simulink model "Exp"  (R2017b)
settings: Solver=FixedStepAuto  StartTime=0.0  StopTime=inf  FixedStep=ts  RelTol=1e-3  EnableMultiTasking=on
values from neighbouring files (symbols this model uses):
  acc_gain = 50    [Init_Exp.m]
  cc = 16    [Init_Exp.m]
  channel = 5    [Init_Exp.m]
  f_gait = 0.1    [Init_Exp.m]
  Kg = 80    [Init_Exp.m]
  R_k = diag([1E-4*[1;1];1E-6*[1;1]])    [Init_Exp.m]
  sigma_p = [0.5 1 100000 100000 100000 100000]'    [Init_Exp.m]
  sigma_pp = [sigma sigma sigma sigma sigma sigma]'    [Init_Exp.m]
  sigma_r = [100000 100000 100000 100000]'    [Init_Exp.m]
  sigma_rr = [sigma sigma sigma sigma]'    [Init_Exp.m]
  systemP = [tau_c2,tau_s2,dqs2,eta2,X2,Y2,J2,tau_c1,tau_s1,dqs1,eta1,X1,Y1,J1]    [Init_Exp.m]
  ts = 0.001    [Init_Exp.m]
  vard = vardtimes*1E-2*[2;1]    [Init_Exp.m]
  vardq = 1E-4*[1;1]    [Init_Exp.m]
  varq = 1E-5*[1;1]    [Init_Exp.m]
undefined symbols (not defined in the file or in its folder): acceleration, command, cxk, desired_acc, desired_position, desired_velocity, DiscIntNeverNeededParam, disturbance, immxk, interaction_force, mkxk, motor_torque, observer, position, velocity, xk
libraries: xpcethercatlib x37, slrtlib x9, simulink x1
(part 1 of 2)
settings Model: xpc_rtwmakecfg_data=_xpcethercatlib_  SimulationMode=external  Creator=Admin  LastModifiedBy=Admin
settings SolverCC: ConcurrentTasks=on  AutoInsertRateTranBlk=on
settings DataIOCC: SaveFormat=StructureWithTime
settings OptimizationCC: BlockReduction=off  OptimizeBlockIOStorage=off  BufferReuse=off  GlobalBufferReuse=off  ExpressionFolding=off  LocalBlockOutputs=off
settings HardwareCC: ProdBitPerPointer=32  ProdBitPerSizeT=32  ProdBitPerPtrDiffT=32  ProdLargestAtomicFloat=None  ProdWordSize=32  ProdLongLongMode=on  ProdHWDeviceType=Generic->32-bit x86 compatible
settings RTWCC: SystemTargetFile=slrt.tlc  TemplateMakefile=slrt_default_tmf  Description=Simulink Real-Time  CodeExecutionProfiling=on  RTWCompilerOptimization=on
settings SimulinkRealTimeCC: SupportVariableSizeSignals=on  RL32LogTETModifier=off  xPCConcurrentTasks=on

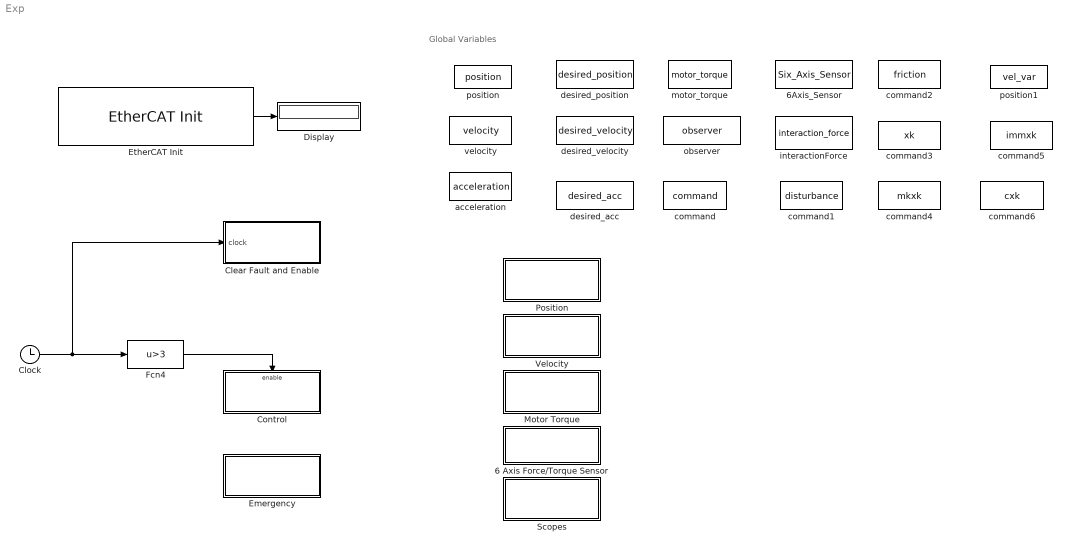
== system Exp ==
  note: Global Variables
  6 Axis Force/Torque Sensor : Subsystem
  6Axis_Sensor : DataStoreMemory  DataStoreName=Six_Axis_Sensor  ReadBeforeWriteMsg=warning  WriteAfterWriteMsg=warning  WriteAfterReadMsg=warning  InitialValue=zeros(12,1)  ShowAdditionalParam=off
  Clear Fault and Enable : Subsystem  TreatAsAtomicUnit=on
  Clock : Clock
  Control : Subsystem  TreatAsAtomicUnit=on
  Display : Display
  Emergency : Subsystem
  "EtherCAT Init " : xpcethercatlib/EtherCAT Init   Priority=0  config_file=D:\lishilei\matlab_workspace\ComputedTorque\GMKMCKF_DOB.xml  device_id=0  pci_bus=2  pci_slot=0  pci_function=0  dctuning=0  enaDebug=off  enaDC=on  errLink=off  masterDbg=off  stateChgDbg=off  baseClock=off  masterCfg=off  logFile='c:\dbglog.txt'  sample_time=0.001000  DCMode=2
      settings: SourceProductName=Simulink Real-Time  SourceProductBaseCode=XP
  Fcn4 : Fcn  Expr=u>3
  Motor Torque : Subsystem
  Position : Subsystem
  Scopes : Subsystem
  Velocity : Subsystem
  acceleration : DataStoreMemory  DataStoreName=acceleration  ReadBeforeWriteMsg=warning  WriteAfterWriteMsg=warning  WriteAfterReadMsg=warning  InitialValue=[0; 0; 0; 0]  ShowAdditionalParam=off
  command : DataStoreMemory  DataStoreName=command  ReadBeforeWriteMsg=warning  WriteAfterWriteMsg=warning  WriteAfterReadMsg=warning  InitialValue=[0; 0; 0; 0]  ShowAdditionalParam=off
  command1 : DataStoreMemory  DataStoreName=disturbance  ReadBeforeWriteMsg=warning  WriteAfterWriteMsg=warning  WriteAfterReadMsg=warning  InitialValue=zeros(4,1)  ShowAdditionalParam=off
  command2 : DataStoreMemory  DataStoreName=friction  ReadBeforeWriteMsg=warning  WriteAfterWriteMsg=warning  WriteAfterReadMsg=warning  InitialValue=[0; 0]  ShowAdditionalParam=off
  command3 : DataStoreMemory  DataStoreName=xk  ReadBeforeWriteMsg=warning  WriteAfterWriteMsg=warning  WriteAfterReadMsg=warning  InitialValue=zeros(6,1)  ShowAdditionalParam=off
  command4 : DataStoreMemory  DataStoreName=mkxk  ReadBeforeWriteMsg=warning  WriteAfterWriteMsg=warning  WriteAfterReadMsg=warning  InitialValue=zeros(6,1)  ShowAdditionalParam=off
  command5 : DataStoreMemory  DataStoreName=immxk  ReadBeforeWriteMsg=warning  WriteAfterWriteMsg=warning  WriteAfterReadMsg=warning  InitialValue=zeros(6,1)  ShowAdditionalParam=off
  command6 : DataStoreMemory  DataStoreName=cxk  ReadBeforeWriteMsg=warning  WriteAfterWriteMsg=warning  WriteAfterReadMsg=warning  InitialValue=zeros(6,1)  ShowAdditionalParam=off
  desired_acc : DataStoreMemory  DataStoreName=desired_acc  ReadBeforeWriteMsg=warning  WriteAfterWriteMsg=warning  WriteAfterReadMsg=warning  InitialValue=[0; 0; 0; 0]  ShowAdditionalParam=off
  desired_position : DataStoreMemory  DataStoreName=desired_position  ReadBeforeWriteMsg=warning  WriteAfterWriteMsg=warning  WriteAfterReadMsg=warning  InitialValue=[0; 0; 0; 0]  ShowAdditionalParam=off
  desired_velocity : DataStoreMemory  DataStoreName=desired_velocity  ReadBeforeWriteMsg=warning  WriteAfterWriteMsg=warning  WriteAfterReadMsg=warning  InitialValue=[0; 0; 0; 0]  ShowAdditionalParam=off
  interactionForce : DataStoreMemory  DataStoreName=interaction_force  ReadBeforeWriteMsg=warning  WriteAfterWriteMsg=warning  WriteAfterReadMsg=warning  InitialValue=[0; 0; 0; 0]  ShowAdditionalParam=off
  motor_torque : DataStoreMemory  DataStoreName=motor_torque  ReadBeforeWriteMsg=warning  WriteAfterWriteMsg=warning  WriteAfterReadMsg=warning  InitialValue=[0; 0; 0; 0]  ShowAdditionalParam=off
  observer : DataStoreMemory  DataStoreName=observer  ReadBeforeWriteMsg=warning  WriteAfterWriteMsg=warning  WriteAfterReadMsg=warning  InitialValue=[0; 0]  ShowAdditionalParam=off
  position : DataStoreMemory  DataStoreName=position  ReadBeforeWriteMsg=warning  WriteAfterWriteMsg=warning  WriteAfterReadMsg=warning  InitialValue=[0; 0; 0; 0]  ShowAdditionalParam=off
  position1 : DataStoreMemory  DataStoreName=vel_var  ReadBeforeWriteMsg=warning  WriteAfterWriteMsg=warning  WriteAfterReadMsg=warning  InitialValue=zeros(2,1)  ShowAdditionalParam=off
  velocity : DataStoreMemory  DataStoreName=velocity  ReadBeforeWriteMsg=warning  WriteAfterWriteMsg=warning  WriteAfterReadMsg=warning  InitialValue=[0; 0; 0; 0]  ShowAdditionalParam=off
  wires:
  Fcn4/1 -> Control/Enable
  Clock/1 -> Clear Fault and Enable/1(clock), Fcn4/1
  "EtherCAT Init "/1 -> Display/1

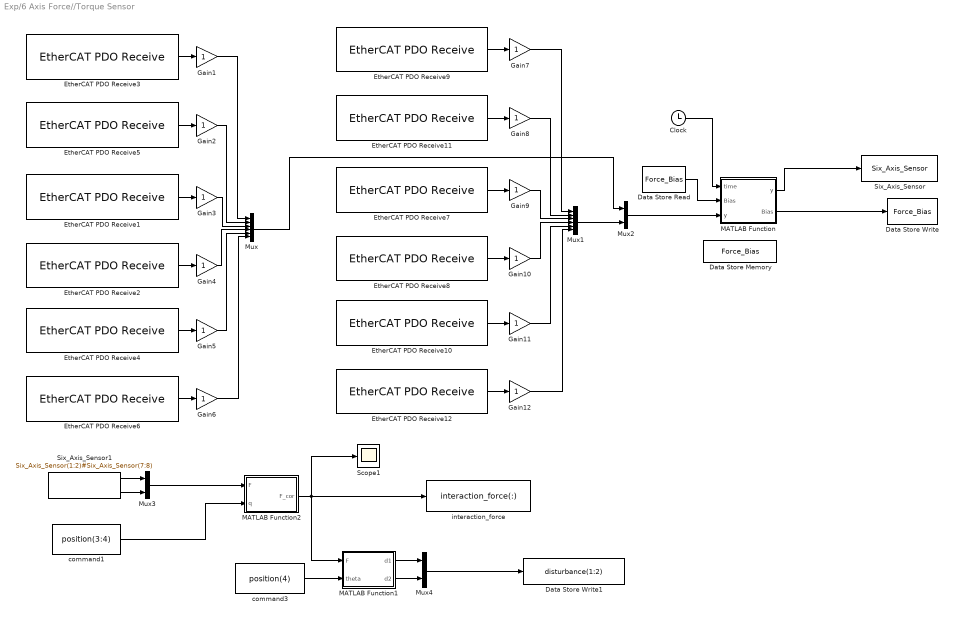
== system Exp/6 Axis Force//Torque Sensor ==
  Clock : Clock
  Data Store Memory : DataStoreMemory  DataStoreName=Force_Bias  ReadBeforeWriteMsg=warning  WriteAfterWriteMsg=warning  WriteAfterReadMsg=warning  InitialValue=zeros(12,1)  ShowAdditionalParam=off
  Data Store Read : DataStoreRead  DataStoreName=Force_Bias
  Data Store Write : DataStoreWrite  DataStoreName=Force_Bias
  Data Store Write1 : DataStoreWrite  DataStoreName=disturbance  DataStoreElements=disturbance(1:2)
  EtherCAT PDO Receive1 : xpcethercatlib/EtherCAT PDO Receive  Priority=2  sig_name=Box 3 (M8126-f32).F/M REAL Inputs.Fz  sig_offset=1160  sig_type=single  type_size=32  sig_dim=1  device_id=0  sample_time=0.001000
      settings: SourceProductName=Simulink Real-Time  SourceProductBaseCode=XP
  EtherCAT PDO Receive10 : xpcethercatlib/EtherCAT PDO Receive  Priority=2  sig_name=Box 4 (M8126-f32).F/M REAL Inputs.My  sig_offset=1432  sig_type=single  type_size=32  sig_dim=1  device_id=0  sample_time=0.001000
      settings: SourceProductName=Simulink Real-Time  SourceProductBaseCode=XP
  EtherCAT PDO Receive11 : xpcethercatlib/EtherCAT PDO Receive  Priority=2  sig_name=Box 4 (M8126-f32).F/M REAL Inputs.Fy  sig_offset=1336  sig_type=single  type_size=32  sig_dim=1  device_id=0  sample_time=0.001000
      settings: SourceProductName=Simulink Real-Time  SourceProductBaseCode=XP
  EtherCAT PDO Receive12 : xpcethercatlib/EtherCAT PDO Receive  Priority=2  sig_name=Box 4 (M8126-f32).F/M REAL Inputs.Mz  sig_offset=1464  sig_type=single  type_size=32  sig_dim=1  device_id=0  sample_time=0.001000
      settings: SourceProductName=Simulink Real-Time  SourceProductBaseCode=XP
  EtherCAT PDO Receive2 : xpcethercatlib/EtherCAT PDO Receive  Priority=2  sig_name=Box 3 (M8126-f32).F/M REAL Inputs.Mx  sig_offset=1192  sig_type=single  type_size=32  sig_dim=1  device_id=0  sample_time=0.001000
      settings: SourceProductName=Simulink Real-Time  SourceProductBaseCode=XP
  EtherCAT PDO Receive3 : xpcethercatlib/EtherCAT PDO Receive  Priority=2  sig_name=Box 3 (M8126-f32).F/M REAL Inputs.Fx  sig_offset=1096  sig_type=single  type_size=32  sig_dim=1  device_id=0  sample_time=0.001000
      settings: SourceProductName=Simulink Real-Time  SourceProductBaseCode=XP
  EtherCAT PDO Receive4 : xpcethercatlib/EtherCAT PDO Receive  Priority=2  sig_name=Box 3 (M8126-f32).F/M REAL Inputs.My  sig_offset=1224  sig_type=single  type_size=32  sig_dim=1  device_id=0  sample_time=0.001000
      settings: SourceProductName=Simulink Real-Time  SourceProductBaseCode=XP
  EtherCAT PDO Receive5 : xpcethercatlib/EtherCAT PDO Receive  Priority=2  sig_name=Box 3 (M8126-f32).F/M REAL Inputs.Fy  sig_offset=1128  sig_type=single  type_size=32  sig_dim=1  device_id=0  sample_time=0.001000
      settings: SourceProductName=Simulink Real-Time  SourceProductBaseCode=XP
  EtherCAT PDO Receive6 : xpcethercatlib/EtherCAT PDO Receive  Priority=2  sig_name=Box 3 (M8126-f32).F/M REAL Inputs.Mz  sig_offset=1256  sig_type=single  type_size=32  sig_dim=1  device_id=0  sample_time=0.001000
      settings: SourceProductName=Simulink Real-Time  SourceProductBaseCode=XP
  EtherCAT PDO Receive7 : xpcethercatlib/EtherCAT PDO Receive  Priority=2  sig_name=Box 4 (M8126-f32).F/M REAL Inputs.Fz  sig_offset=1368  sig_type=single  type_size=32  sig_dim=1  device_id=0  sample_time=0.001000
      settings: SourceProductName=Simulink Real-Time  SourceProductBaseCode=XP
  EtherCAT PDO Receive8 : xpcethercatlib/EtherCAT PDO Receive  Priority=2  sig_name=Box 4 (M8126-f32).F/M REAL Inputs.Mx  sig_offset=1400  sig_type=single  type_size=32  sig_dim=1  device_id=0  sample_time=0.001000
      settings: SourceProductName=Simulink Real-Time  SourceProductBaseCode=XP
  EtherCAT PDO Receive9 : xpcethercatlib/EtherCAT PDO Receive  Priority=2  sig_name=Box 4 (M8126-f32).F/M REAL Inputs.Fx  sig_offset=1304  sig_type=single  type_size=32  sig_dim=1  device_id=0  sample_time=0.001000
      settings: SourceProductName=Simulink Real-Time  SourceProductBaseCode=XP
  Gain{1..12} (12 alike) : Gain  OutDataTypeStr=double
  MATLAB Function : MATLAB Function  TreatAsAtomicUnit=on
  MATLAB Function1 : MATLAB Function  TreatAsAtomicUnit=on
  MATLAB Function2 : MATLAB Function  TreatAsAtomicUnit=on
  Mux : Mux  Inputs=6
  Mux1 : Mux  Inputs=6
  Mux2 : Mux  Inputs=2
  Mux3 : Mux  Inputs=2
  Mux4 : Mux  Inputs=2
  Scope1 : Scope
  Six_Axis_Sensor : DataStoreWrite  DataStoreName=Six_Axis_Sensor
  Six_Axis_Sensor1 : DataStoreRead  DataStoreName=Six_Axis_Sensor  DataStoreElements=Six_Axis_Sensor(1:2)#Six_Axis_Sensor(7:8)
  command1 : DataStoreRead  DataStoreName=position  DataStoreElements=position(3:4)
  command3 : DataStoreRead  DataStoreName=position  DataStoreElements=position(4)
  interaction_force : DataStoreWrite  DataStoreName=interaction_force  DataStoreElements=interaction_force(:)
  wires:
  Gain3/1 -> Mux/3
  EtherCAT PDO Receive5/1 -> Gain2/1
  EtherCAT PDO Receive3/1 -> Gain1/1
  Gain4/1 -> Mux/4
  EtherCAT PDO Receive4/1 -> Gain5/1
  EtherCAT PDO Receive6/1 -> Gain6/1
  Mux/1 -> Mux2/1
  Clock/1 -> MATLAB Function/1(time)
  Mux2/1 -> MATLAB Function/3("y ")
  Data Store Read/1 -> MATLAB Function/2("Bias ")
  MATLAB Function/2(Bias) -> Data Store Write/1
  MATLAB Function/1(y) -> Six_Axis_Sensor/1
  EtherCAT PDO Receive12/1 -> Gain12/1
  EtherCAT PDO Receive11/1 -> Gain8/1
  EtherCAT PDO Receive8/1 -> Gain10/1
  EtherCAT PDO Receive10/1 -> Gain11/1
  EtherCAT PDO Receive7/1 -> Gain9/1
  Mux1/1 -> Mux2/2
  EtherCAT PDO Receive9/1 -> Gain7/1
  Gain1/1 -> Mux/1
  Gain2/1 -> Mux/2
  EtherCAT PDO Receive1/1 -> Gain3/1
  EtherCAT PDO Receive2/1 -> Gain4/1
  Gain5/1 -> Mux/5
  Gain6/1 -> Mux/6
  Gain7/1 -> Mux1/1
  Gain8/1 -> Mux1/2
  Gain9/1 -> Mux1/3
  Gain10/1 -> Mux1/4
  Gain11/1 -> Mux1/5
  Gain12/1 -> Mux1/6
  MATLAB Function2/1(F_cor) -> Scope1/1, MATLAB Function1/1(F), interaction_force/1
  command3/1 -> MATLAB Function1/2(theta)
  Mux4/1 -> Data Store Write1/1
  MATLAB Function1/1(d1) -> Mux4/1
  MATLAB Function1/2(d2) -> Mux4/2
  Six_Axis_Sensor1/1 -> Mux3/1
  Six_Axis_Sensor1/2 -> Mux3/2
  Mux3/1 -> MATLAB Function2/1(F)
  command1/1 -> MATLAB Function2/2(q)

== system Exp/Clear Fault and Enable ==
  clock : Inport
  Enable 1 : Subsystem  TreatAsAtomicUnit=on
  Enable 2 : Subsystem  TreatAsAtomicUnit=on
  Fcn1 : Fcn  Expr=u<2.5
  Fcn5 : Fcn  Expr=u<3&&u>2.5
  wires:
  Fcn5/1 -> Enable 2/Enable
  Fcn1/1 -> Enable 1/Enable
  clock/1 -> Fcn5/1, Fcn1/1

== system Exp/Control ==
  Enable : EnablePort
  Execution : Subsystem
  Feedforward&nonlinearFeekbackLinearlization&Observer : Subsystem
  Gait Generator : Subsystem
  PD controller : Subsystem

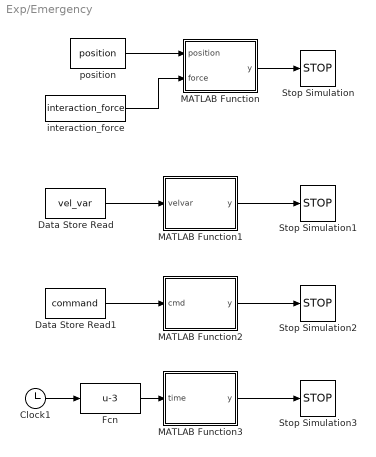
== system Exp/Emergency ==
  Clock1 : Clock
  Data Store Read : DataStoreRead  DataStoreName=vel_var
  Data Store Read1 : DataStoreRead  DataStoreName=command
  Fcn : Fcn  Expr=u-3
  MATLAB Function : MATLAB Function  TreatAsAtomicUnit=on
  MATLAB Function1 : MATLAB Function  TreatAsAtomicUnit=on
  MATLAB Function2 : MATLAB Function  TreatAsAtomicUnit=on
  MATLAB Function3 : MATLAB Function  TreatAsAtomicUnit=on
  Stop Simulation{,1..3} (4 alike) : Stop
  interaction_force : DataStoreRead  DataStoreName=interaction_force
  position : DataStoreRead  DataStoreName=position
  wires:
  position/1 -> MATLAB Function/1(position)
  MATLAB Function/1(y) -> Stop Simulation/1
  interaction_force/1 -> MATLAB Function/2(force)
  Data Store Read/1 -> MATLAB Function1/1(velvar)
  MATLAB Function1/1(y) -> Stop Simulation1/1
  Data Store Read1/1 -> MATLAB Function2/1(cmd)
  MATLAB Function2/1(y) -> Stop Simulation2/1
  Clock1/1 -> Fcn/1
  Fcn/1 -> MATLAB Function3/1(time)
  MATLAB Function3/1(y) -> Stop Simulation3/1

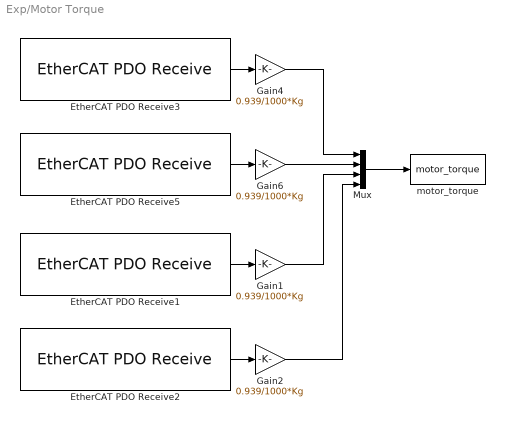
== system Exp/Motor Torque ==
  EtherCAT PDO Receive1 : xpcethercatlib/EtherCAT PDO Receive  Priority=2  sig_name=Drive 2 (AE2).Module 1 (Cyclic torque Mode).Cyclic torque Inputs.Torque actual value  sig_offset=936  sig_type=int16  type_size=16  sig_dim=1  device_id=0  sample_time=0.001000
      settings: SourceProductName=Simulink Real-Time  SourceProductBaseCode=XP
  EtherCAT PDO Receive2 : xpcethercatlib/EtherCAT PDO Receive  Priority=2  sig_name=Drive 2 (AE2).Module 2 (Cyclic torque Mode).Cyclic torque Inputs.Torque actual value  sig_offset=1064  sig_type=int16  type_size=16  sig_dim=1  device_id=0  sample_time=0.001000
      settings: SourceProductName=Simulink Real-Time  SourceProductBaseCode=XP
  EtherCAT PDO Receive3 : xpcethercatlib/EtherCAT PDO Receive  Priority=2  sig_name=Drive 1 (AE2).Module 1 (Cyclic torque Mode).Cyclic torque Inputs.Torque actual value  sig_offset=680  sig_type=int16  type_size=16  sig_dim=1  device_id=0  sample_time=0.001000
      settings: SourceProductName=Simulink Real-Time  SourceProductBaseCode=XP
  EtherCAT PDO Receive5 : xpcethercatlib/EtherCAT PDO Receive  Priority=2  sig_name=Drive 1 (AE2).Module 2 (Cyclic torque Mode).Cyclic torque Inputs.Torque actual value  sig_offset=808  sig_type=int16  type_size=16  sig_dim=1  device_id=0  sample_time=0.001000
      settings: SourceProductName=Simulink Real-Time  SourceProductBaseCode=XP
  Gain{1..2,4,6} (4 alike) : Gain  Gain=0.939/1000*Kg  OutDataTypeStr=double
  Mux : Mux
  motor_torque : DataStoreWrite  DataStoreName=motor_torque
  wires:
  EtherCAT PDO Receive3/1 -> Gain4/1
  EtherCAT PDO Receive5/1 -> Gain6/1
  EtherCAT PDO Receive1/1 -> Gain1/1
  EtherCAT PDO Receive2/1 -> Gain2/1
  Mux/1 -> motor_torque/1
  Gain6/1 -> Mux/2
  Gain1/1 -> Mux/3
  Gain2/1 -> Mux/4
  Gain4/1 -> Mux/1

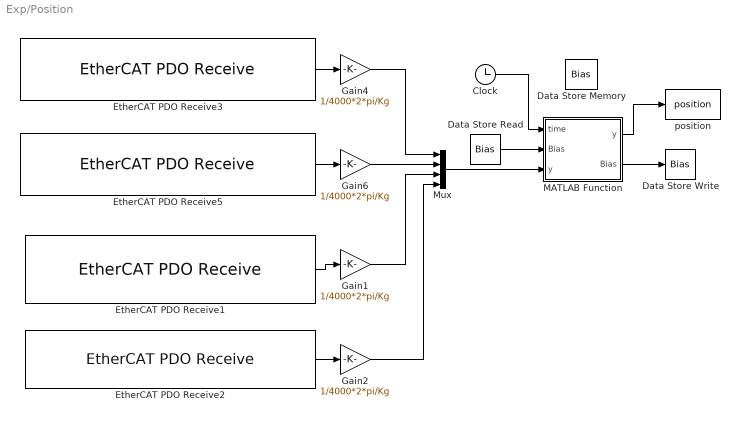
== system Exp/Position ==
  Clock : Clock
  Data Store Memory : DataStoreMemory  DataStoreName=Bias  ReadBeforeWriteMsg=warning  WriteAfterWriteMsg=warning  WriteAfterReadMsg=warning  InitialValue=zeros(4,1)  ShowAdditionalParam=off
  Data Store Read : DataStoreRead  DataStoreName=Bias
  Data Store Write : DataStoreWrite  DataStoreName=Bias
  EtherCAT PDO Receive1 : xpcethercatlib/EtherCAT PDO Receive  Priority=2  sig_name=Drive 2 (AE2).Module 1 (Cyclic torque Mode).Cyclic torque Inputs.Actual motor position  sig_offset=840  sig_type=int32  type_size=32  sig_dim=1  device_id=0  sample_time=0.001000
      settings: SourceProductName=Simulink Real-Time  SourceProductBaseCode=XP
  EtherCAT PDO Receive2 : xpcethercatlib/EtherCAT PDO Receive  Priority=2  sig_name=Drive 2 (AE2).Module 2 (Cyclic torque Mode).Cyclic torque Inputs.Actual motor position  sig_offset=968  sig_type=int32  type_size=32  sig_dim=1  device_id=0  sample_time=0.001000
      settings: SourceProductName=Simulink Real-Time  SourceProductBaseCode=XP
  EtherCAT PDO Receive3 : xpcethercatlib/EtherCAT PDO Receive  Priority=2  sig_name=Drive 1 (AE2).Module 1 (Cyclic torque Mode).Cyclic torque Inputs.Actual motor position  sig_offset=584  sig_type=int32  type_size=32  sig_dim=1  device_id=0  sample_time=0.001000
      settings: SourceProductName=Simulink Real-Time  SourceProductBaseCode=XP
  EtherCAT PDO Receive5 : xpcethercatlib/EtherCAT PDO Receive  Priority=2  sig_name=Drive 1 (AE2).Module 2 (Cyclic torque Mode).Cyclic torque Inputs.Actual motor position  sig_offset=712  sig_type=int32  type_size=32  sig_dim=1  device_id=0  sample_time=0.001000
      settings: SourceProductName=Simulink Real-Time  SourceProductBaseCode=XP
  Gain{1..2,4,6} (4 alike) : Gain  Gain=1/4000*2*pi/Kg  OutDataTypeStr=double
  MATLAB Function : MATLAB Function  TreatAsAtomicUnit=on
  Mux : Mux
  position : DataStoreWrite  DataStoreName=position
  wires:
  EtherCAT PDO Receive3/1 -> Gain4/1
  EtherCAT PDO Receive5/1 -> Gain6/1
  Gain4/1 -> Mux/1
  Gain6/1 -> Mux/2
  EtherCAT PDO Receive1/1 -> Gain1/1
  EtherCAT PDO Receive2/1 -> Gain2/1
  Gain1/1 -> Mux/3
  Gain2/1 -> Mux/4
  Mux/1 -> MATLAB Function/3("y ")
  Clock/1 -> MATLAB Function/1(time)
  Data Store Read/1 -> MATLAB Function/2("Bias ")
  MATLAB Function/2(Bias) -> Data Store Write/1
  MATLAB Function/1(y) -> position/1

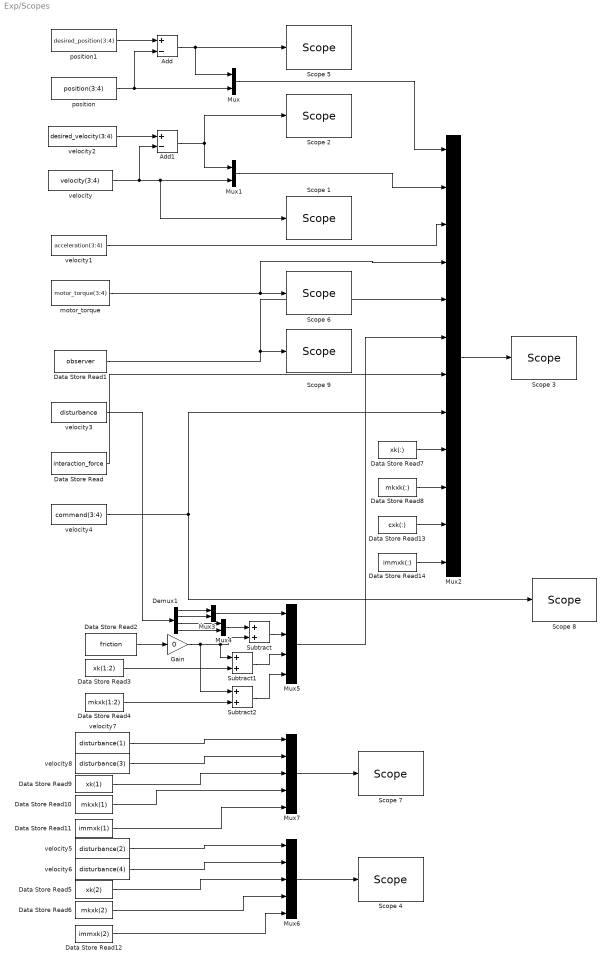
== system Exp/Scopes ==
  Add : Sum  Inputs=+-
  Add1 : Sum  Inputs=+-
  Data Store Read : DataStoreRead  DataStoreName=interaction_force
  Data Store Read1 : DataStoreRead  DataStoreName=observer
  Data Store Read10 : DataStoreRead  DataStoreName=mkxk  DataStoreElements=mkxk(1)
  Data Store Read11 : DataStoreRead  DataStoreName=immxk  DataStoreElements=immxk(1)
  Data Store Read12 : DataStoreRead  DataStoreName=immxk  DataStoreElements=immxk(2)
  Data Store Read13 : DataStoreRead  DataStoreName=cxk  DataStoreElements=cxk(:)
  Data Store Read14 : DataStoreRead  DataStoreName=immxk  DataStoreElements=immxk(:)
  Data Store Read2 : DataStoreRead  DataStoreName=friction
  Data Store Read3 : DataStoreRead  DataStoreName=xk  DataStoreElements=xk(1:2)
  Data Store Read4 : DataStoreRead  DataStoreName=mkxk  DataStoreElements=mkxk(1:2)
  Data Store Read5 : DataStoreRead  DataStoreName=xk  DataStoreElements=xk(2)
  Data Store Read6 : DataStoreRead  DataStoreName=mkxk  DataStoreElements=mkxk(2)
  Data Store Read7 : DataStoreRead  DataStoreName=xk  DataStoreElements=xk(:)
  Data Store Read8 : DataStoreRead  DataStoreName=mkxk  DataStoreElements=mkxk(:)
  Data Store Read9 : DataStoreRead  DataStoreName=xk  DataStoreElements=xk(1)
  Demux1 : Demux
  Gain : Gain  Gain=0
  Mux{,1,3..4} (4 alike) : Mux  Inputs=2
  Mux2 : Mux  Inputs=12
  Mux5 : Mux
  Mux6 : Mux  Inputs=5
  Mux7 : Mux  Inputs=5
  Scope 1 : slrtlib/Displays and Logging/Scope   scopeno=3  scopetype=Target  autostart=on  viewmode=Graphical sliding  formatstr='%15.6f'  grid=on  ylimits=[-1.5, 1.5]  nosamples=10/ts  noprepostsamples=0  interleave=1  triggermode=FreeRun  triggersignal=1  trigsignalfromport=off  triggerlevel=0.0  triggerslope=Either  triggerscope=1  triggersample=0  filename=data.dat  mode=Lazy  writesize=512  autorestart=off  dynamicfilemode=off  maxwritefilesize=512*1024^2
  Scope 2 : slrtlib/Displays and Logging/Scope   scopeno=2  scopetype=Target  autostart=on  viewmode=Graphical sliding  formatstr='%15.6f'  grid=on  ylimits=[-0.2, 0.2]  nosamples=10/ts  noprepostsamples=0  interleave=1  triggermode=FreeRun  triggersignal=1  trigsignalfromport=off  triggerlevel=0.0  triggerslope=Either  triggerscope=1  triggersample=0  filename=data.dat  mode=Lazy  writesize=512  autorestart=off  dynamicfilemode=off  maxwritefilesize=512*1024^2
  Scope 3 : slrtlib/Displays and Logging/Scope   scopeno=9  scopetype=File  autostart=on  viewmode=Graphical sliding  formatstr='%15.6f'  grid=on  ylimits=[-1.5, 1.5]  nosamples=1000000  noprepostsamples=0  interleave=1  triggermode=FreeRun  triggersignal=1  trigsignalfromport=off  triggerlevel=0.0  triggerslope=Either  triggerscope=1  triggersample=0  filename=exp_data.dat  mode=Lazy  writesize=512  autorestart=off  dynamicfilemode=off  maxwritefilesize=512*1024^2
  Scope 4 : slrtlib/Displays and Logging/Scope   scopeno=7  scopetype=Target  autostart=on  viewmode=Graphical sliding  formatstr='%15.6f'  grid=on  ylimits=[-40, 40]  nosamples=10/ts  noprepostsamples=0  interleave=1  triggermode=FreeRun  triggersignal=1  trigsignalfromport=off  triggerlevel=0.0  triggerslope=Either  triggerscope=1  triggersample=0  filename=data.dat  mode=Lazy  writesize=512  autorestart=off  dynamicfilemode=off  maxwritefilesize=512*1024^2
  Scope 5 : slrtlib/Displays and Logging/Scope   scopeno=1  scopetype=Target  autostart=on  viewmode=Graphical sliding  formatstr='%15.6f'  grid=on  ylimits=[-0.005, 0.005]  nosamples=10/ts  noprepostsamples=0  interleave=1  triggermode=FreeRun  triggersignal=1  trigsignalfromport=off  triggerlevel=0.0  triggerslope=Either  triggerscope=1  triggersample=0  filename=data.dat  mode=Lazy  writesize=512  autorestart=off  dynamicfilemode=off  maxwritefilesize=512*1024^2
  Scope 6 : slrtlib/Displays and Logging/Scope   scopeno=4  scopetype=Target  autostart=on  viewmode=Graphical sliding  formatstr='%15.6f'  grid=on  ylimits=[-30, 30]  nosamples=10/ts  noprepostsamples=0  interleave=1  triggermode=FreeRun  triggersignal=1  trigsignalfromport=off  triggerlevel=0.0  triggerslope=Either  triggerscope=1  triggersample=0  filename=data.dat  mode=Lazy  writesize=512  autorestart=off  dynamicfilemode=off  maxwritefilesize=512*1024^2
  Scope 7 : slrtlib/Displays and Logging/Scope   scopeno=6  scopetype=Target  autostart=on  viewmode=Graphical sliding  formatstr='%15.6f'  grid=on  ylimits=[-40, 40]  nosamples=10/ts  noprepostsamples=0  interleave=1  triggermode=FreeRun  triggersignal=1  trigsignalfromport=off  triggerlevel=0.0  triggerslope=Either  triggerscope=1  triggersample=0  filename=data.dat  mode=Lazy  writesize=512  autorestart=off  dynamicfilemode=off  maxwritefilesize=512*1024^2
  Scope 8 : slrtlib/Displays and Logging/Scope   scopeno=8  scopetype=Target  autostart=on  viewmode=Graphical sliding  formatstr='%15.6f'  grid=on  ylimits=[-50, 50]  nosamples=10/ts  noprepostsamples=0  interleave=1  triggermode=FreeRun  triggersignal=1  trigsignalfromport=off  triggerlevel=0.0  triggerslope=Either  triggerscope=1  triggersample=0  filename=data.dat  mode=Lazy  writesize=512  autorestart=off  dynamicfilemode=off  maxwritefilesize=512*1024^2
  Scope 9 : slrtlib/Displays and Logging/Scope   scopeno=5  scopetype=Target  autostart=on  viewmode=Graphical sliding  formatstr='%15.6f'  grid=on  ylimits=[-30, 30]  nosamples=10/ts  noprepostsamples=0  interleave=1  triggermode=FreeRun  triggersignal=1  trigsignalfromport=off  triggerlevel=0.0  triggerslope=Either  triggerscope=1  triggersample=0  filename=data.dat  mode=Lazy  writesize=512  autorestart=off  dynamicfilemode=off  maxwritefilesize=512*1024^2
  Subtract : Sum
  Subtract1 : Sum
  Subtract2 : Sum
  motor_torque : DataStoreRead  DataStoreName=motor_torque  DataStoreElements=motor_torque(3:4)
  position : DataStoreRead  DataStoreName=position  DataStoreElements=position(3:4)
  position1 : DataStoreRead  DataStoreName=desired_position  DataStoreElements=desired_position(3:4)
  velocity : DataStoreRead  DataStoreName=velocity  DataStoreElements=velocity(3:4)
  velocity1 : DataStoreRead  DataStoreName=acceleration  DataStoreElements=acceleration(3:4)
  velocity2 : DataStoreRead  DataStoreName=desired_velocity  DataStoreElements=desired_velocity(3:4)
  velocity3 : DataStoreRead  DataStoreName=disturbance
  velocity4 : DataStoreRead  DataStoreName=command  DataStoreElements=command(3:4)
  velocity5 : DataStoreRead  DataStoreName=disturbance  DataStoreElements=disturbance(2)
  velocity6 : DataStoreRead  DataStoreName=disturbance  DataStoreElements=disturbance(4)
  velocity7 : DataStoreRead  DataStoreName=disturbance  DataStoreElements=disturbance(1)
  velocity8 : DataStoreRead  DataStoreName=disturbance  DataStoreElements=disturbance(3)
  wires:
  velocity/1 -> Add1/2, Scope 1/1, Mux1/2
  motor_torque/1 -> Mux2/4, Scope 6/1
  Mux2/1 -> Scope 3/1
  position/1 -> Mux/2, Add/2
  position1/1 -> Add/1
  velocity2/1 -> Add1/1
  Add/1 -> Mux/1, Scope 5/1
  Add1/1 -> Scope 2/1, Mux1/1
  Mux/1 -> Mux2/1
  Mux1/1 -> Mux2/2
  velocity1/1 -> Mux2/3
  Data Store Read1/1 -> Scope 9/1, Mux2/5
  velocity3/1 -> Demux1/1
  Data Store Read/1 -> Mux2/7
  velocity4/1 -> Mux2/8, Scope 8/1
  Demux1/1 -> Mux3/1
  Demux1/2 -> Mux3/2
  Demux1/3 -> Mux4/1
  Demux1/4 -> Mux4/2
  Mux4/1 -> Subtract/1
  Data Store Read2/1 -> Gain/1
  Subtract/1 -> Mux5/2
  Mux3/1 -> Mux5/1
  Mux5/1 -> Mux2/6
  Gain/1 -> Subtract2/1, Subtract1/1, Subtract/2
  velocity5/1 -> Mux6/1
  velocity6/1 -> Mux6/2
  Data Store Read5/1 -> Mux6/3
  Data Store Read6/1 -> Mux6/4
  Mux6/1 -> Scope 4/1
  Data Store Read8/1 -> Mux2/10
  Data Store Read7/1 -> Mux2/9
  Data Store Read4/1 -> Subtract2/2
  Subtract2/1 -> Mux5/4
  Data Store Read3/1 -> Subtract1/2
  Subtract1/1 -> Mux5/3
  Data Store Read9/1 -> Mux7/3
  velocity7/1 -> Mux7/1
  velocity8/1 -> Mux7/2
  Mux7/1 -> Scope 7/1
  Data Store Read10/1 -> Mux7/4
  Data Store Read11/1 -> Mux7/5
  Data Store Read12/1 -> Mux6/5
  Data Store Read13/1 -> Mux2/11
  Data Store Read14/1 -> Mux2/12

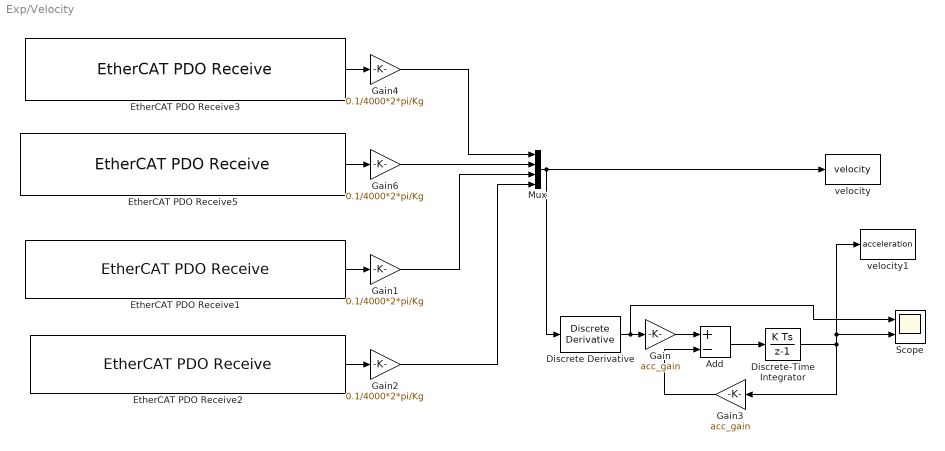
== system Exp/Velocity ==
  Add : Sum  Inputs=+-
  Discrete Derivative : simulink/Discrete/Discrete Derivative  gainval=1.0  ICPrevScaledInput=0.0  OutMin=[]  OutMax=[]  OutDataType=fixdt(1, 16)  OutScaling=2^-10  DoSatur=off
  Discrete-Time Integrator : DiscreteIntegrator  InitialConditionSetting=State (most efficient)  SampleTime=ts  ICPrevOutput=DiscIntNeverNeededParam  ICPrevScaledInput=DiscIntNeverNeededParam
  EtherCAT PDO Receive1 : xpcethercatlib/EtherCAT PDO Receive  Priority=2  sig_name=Drive 2 (AE2).Module 1 (Cyclic torque Mode).Cyclic torque Inputs.Actual motor velocity  sig_offset=904  sig_type=int32  type_size=32  sig_dim=1  device_id=0  sample_time=0.001000
      settings: SourceProductName=Simulink Real-Time  SourceProductBaseCode=XP
  EtherCAT PDO Receive2 : xpcethercatlib/EtherCAT PDO Receive  Priority=2  sig_name=Drive 2 (AE2).Module 2 (Cyclic torque Mode).Cyclic torque Inputs.Actual motor velocity  sig_offset=1032  sig_type=int32  type_size=32  sig_dim=1  device_id=0  sample_time=0.001000
      settings: SourceProductName=Simulink Real-Time  SourceProductBaseCode=XP
  EtherCAT PDO Receive3 : xpcethercatlib/EtherCAT PDO Receive  Priority=2  sig_name=Drive 1 (AE2).Module 1 (Cyclic torque Mode).Cyclic torque Inputs.Actual motor velocity  sig_offset=648  sig_type=int32  type_size=32  sig_dim=1  device_id=0  sample_time=0.001000
      settings: SourceProductName=Simulink Real-Time  SourceProductBaseCode=XP
  EtherCAT PDO Receive5 : xpcethercatlib/EtherCAT PDO Receive  Priority=2  sig_name=Drive 1 (AE2).Module 2 (Cyclic torque Mode).Cyclic torque Inputs.Actual motor velocity  sig_offset=776  sig_type=int32  type_size=32  sig_dim=1  device_id=0  sample_time=0.001000
      settings: SourceProductName=Simulink Real-Time  SourceProductBaseCode=XP
  Gain : Gain  Gain=acc_gain
  Gain{1..2,4,6} (4 alike) : Gain  Gain=0.1/4000*2*pi/Kg  OutDataTypeStr=double
  Gain3 : Gain  Gain=acc_gain
  Mux : Mux
  Scope : Scope  NumInputPorts=2
  velocity : DataStoreWrite  DataStoreName=velocity
  velocity1 : DataStoreWrite  DataStoreName=acceleration
  wires:
  EtherCAT PDO Receive3/1 -> Gain4/1
  EtherCAT PDO Receive5/1 -> Gain6/1
  EtherCAT PDO Receive2/1 -> Gain2/1
  EtherCAT PDO Receive1/1 -> Gain1/1
  Gain2/1 -> Mux/4
  Gain1/1 -> Mux/3
  Gain4/1 -> Mux/1
  Gain6/1 -> Mux/2
  Mux/1 -> velocity/1, Discrete Derivative/1
  Add/1 -> Discrete-Time Integrator/1
  Gain/1 -> Add/1
  Discrete-Time Integrator/1 -> Gain3/1, Scope/2, velocity1/1
  Gain3/1 -> Add/2
  Discrete Derivative/1 -> Scope/1, Gain/1

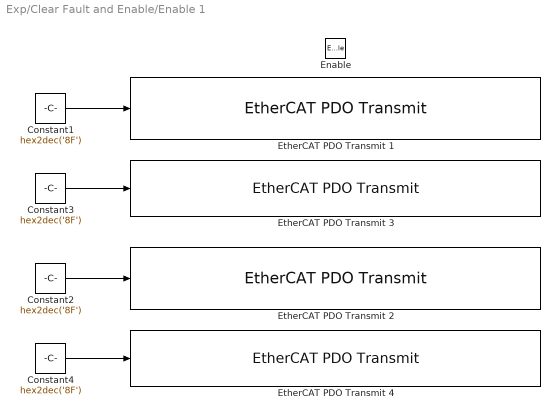
== system Exp/Clear Fault and Enable/Enable 1 ==
  Enable : EnablePort
  Constant{1..4} (4 alike) : Constant  Value=hex2dec('8F')  OutDataTypeStr=uint16
  EtherCAT PDO Transmit 1 : xpcethercatlib/EtherCAT PDO Transmit   Priority=3  sig_name=Drive 1 (AE2).Module 1 (Cyclic torque Mode).Cyclic torque Outputs.Control word  sig_offset=568  sig_type=uint16  type_size=16  sig_dim=1  device_id=0  sample_time=0.001000
      settings: SourceProductName=Simulink Real-Time  SourceProductBaseCode=XP
  EtherCAT PDO Transmit 2 : xpcethercatlib/EtherCAT PDO Transmit   Priority=3  sig_name=Drive 2 (AE2).Module 1 (Cyclic torque Mode).Cyclic torque Outputs.Control word  sig_offset=824  sig_type=uint16  type_size=16  sig_dim=1  device_id=0  sample_time=0.001000
      settings: SourceProductName=Simulink Real-Time  SourceProductBaseCode=XP
  EtherCAT PDO Transmit 3 : xpcethercatlib/EtherCAT PDO Transmit   Priority=3  sig_name=Drive 1 (AE2).Module 2 (Cyclic torque Mode).Cyclic torque Outputs.Control word  sig_offset=600  sig_type=uint16  type_size=16  sig_dim=1  device_id=0  sample_time=0.001000
      settings: SourceProductName=Simulink Real-Time  SourceProductBaseCode=XP
  EtherCAT PDO Transmit 4 : xpcethercatlib/EtherCAT PDO Transmit   Priority=3  sig_name=Drive 2 (AE2).Module 2 (Cyclic torque Mode).Cyclic torque Outputs.Control word  sig_offset=856  sig_type=uint16  type_size=16  sig_dim=1  device_id=0  sample_time=0.001000
      settings: SourceProductName=Simulink Real-Time  SourceProductBaseCode=XP
  wires:
  Constant1/1 -> EtherCAT PDO Transmit 1/1
  Constant3/1 -> EtherCAT PDO Transmit 3/1
  Constant2/1 -> EtherCAT PDO Transmit 2/1
  Constant4/1 -> EtherCAT PDO Transmit 4/1

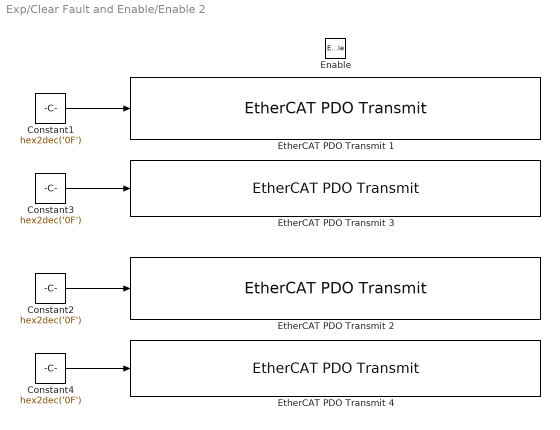
== system Exp/Clear Fault and Enable/Enable 2 ==
  Enable : EnablePort
  Constant{1..4} (4 alike) : Constant  Value=hex2dec('0F')  OutDataTypeStr=uint16
  EtherCAT PDO Transmit 1 : xpcethercatlib/EtherCAT PDO Transmit   Priority=3  sig_name=Drive 1 (AE2).Module 1 (Cyclic torque Mode).Cyclic torque Outputs.Control word  sig_offset=568  sig_type=uint16  type_size=16  sig_dim=1  device_id=0  sample_time=0.001000
      settings: SourceProductName=Simulink Real-Time  SourceProductBaseCode=XP
  EtherCAT PDO Transmit 2 : xpcethercatlib/EtherCAT PDO Transmit   Priority=3  sig_name=Drive 2 (AE2).Module 1 (Cyclic torque Mode).Cyclic torque Outputs.Control word  sig_offset=824  sig_type=uint16  type_size=16  sig_dim=1  device_id=0  sample_time=0.001000
      settings: SourceProductName=Simulink Real-Time  SourceProductBaseCode=XP
  EtherCAT PDO Transmit 3 : xpcethercatlib/EtherCAT PDO Transmit   Priority=3  sig_name=Drive 1 (AE2).Module 2 (Cyclic torque Mode).Cyclic torque Outputs.Control word  sig_offset=600  sig_type=uint16  type_size=16  sig_dim=1  device_id=0  sample_time=0.001000
      settings: SourceProductName=Simulink Real-Time  SourceProductBaseCode=XP
  EtherCAT PDO Transmit 4 : xpcethercatlib/EtherCAT PDO Transmit   Priority=3  sig_name=Drive 2 (AE2).Module 2 (Cyclic torque Mode).Cyclic torque Outputs.Control word  sig_offset=856  sig_type=uint16  type_size=16  sig_dim=1  device_id=0  sample_time=0.001000
      settings: SourceProductName=Simulink Real-Time  SourceProductBaseCode=XP
  wires:
  Constant1/1 -> EtherCAT PDO Transmit 1/1
  Constant3/1 -> EtherCAT PDO Transmit 3/1
  Constant4/1 -> EtherCAT PDO Transmit 4/1
  Constant2/1 -> EtherCAT PDO Transmit 2/1

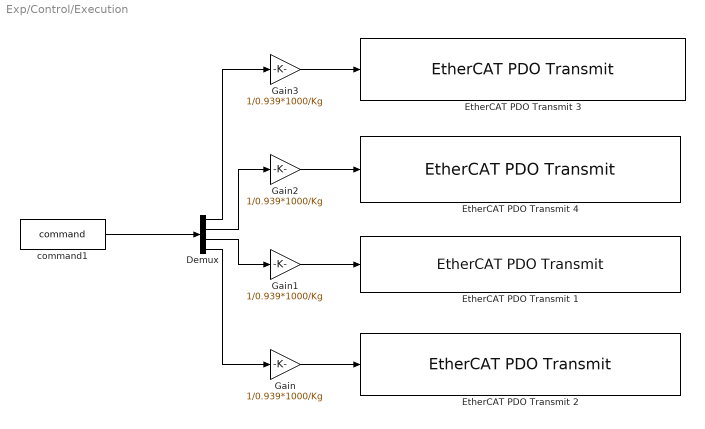
== system Exp/Control/Execution ==
  Demux : Demux
  EtherCAT PDO Transmit 1 : xpcethercatlib/EtherCAT PDO Transmit   Priority=3  sig_name=Drive 2 (AE2).Module 1 (Cyclic torque Mode).Cyclic torque Outputs.Target Torque  sig_offset=840  sig_type=int16  type_size=16  sig_dim=1  device_id=0  sample_time=0.001000
      settings: SourceProductName=Simulink Real-Time  SourceProductBaseCode=XP
  EtherCAT PDO Transmit 2 : xpcethercatlib/EtherCAT PDO Transmit   Priority=3  sig_name=Drive 2 (AE2).Module 2 (Cyclic torque Mode).Cyclic torque Outputs.Target Torque  sig_offset=872  sig_type=int16  type_size=16  sig_dim=1  device_id=0  sample_time=0.001000
      settings: SourceProductName=Simulink Real-Time  SourceProductBaseCode=XP
  EtherCAT PDO Transmit 3 : xpcethercatlib/EtherCAT PDO Transmit   Priority=3  sig_name=Drive 1 (AE2).Module 1 (Cyclic torque Mode).Cyclic torque Outputs.Target Torque  sig_offset=584  sig_type=int16  type_size=16  sig_dim=1  device_id=0  sample_time=0.001000
      settings: SourceProductName=Simulink Real-Time  SourceProductBaseCode=XP
  EtherCAT PDO Transmit 4 : xpcethercatlib/EtherCAT PDO Transmit   Priority=3  sig_name=Drive 1 (AE2).Module 2 (Cyclic torque Mode).Cyclic torque Outputs.Target Torque  sig_offset=616  sig_type=int16  type_size=16  sig_dim=1  device_id=0  sample_time=0.001000
      settings: SourceProductName=Simulink Real-Time  SourceProductBaseCode=XP
  Gain{,1..3} (4 alike) : Gain  Gain=1/0.939*1000/Kg  OutDataTypeStr=int16
  command1 : DataStoreRead  DataStoreName=command
  wires:
  Demux/1 -> Gain3/1
  Demux/3 -> Gain1/1
  Gain3/1 -> EtherCAT PDO Transmit 3/1
  Gain1/1 -> EtherCAT PDO Transmit 1/1
  Gain/1 -> EtherCAT PDO Transmit 2/1
  Demux/2 -> Gain2/1
  Demux/4 -> Gain/1
  command1/1 -> Demux/1
  Gain2/1 -> EtherCAT PDO Transmit 4/1

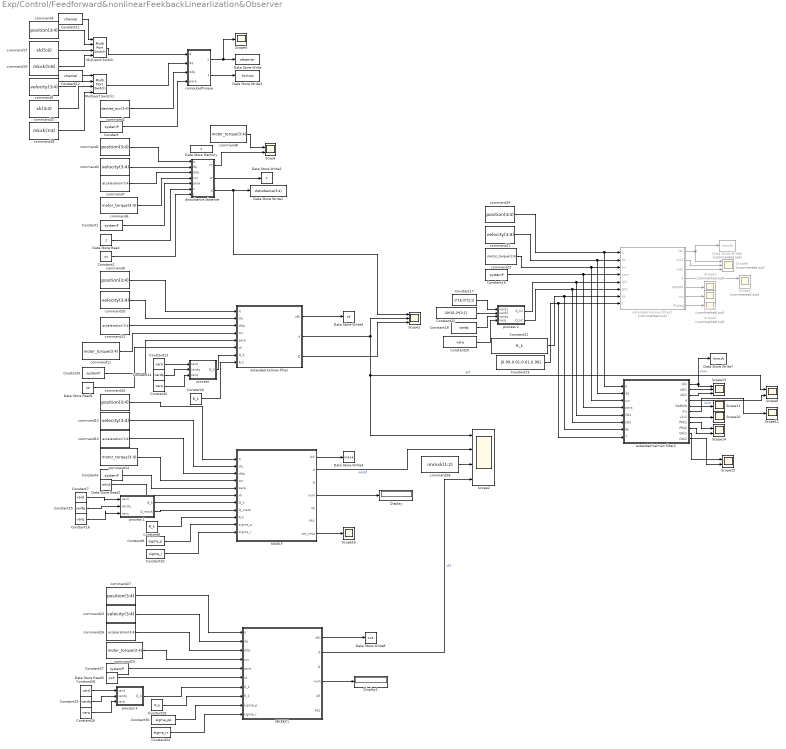
== system Exp/Control/Feedforward&nonlinearFeekbackLinearlization&Observer ==
  Constant{,1,3..4,19,27} (6 alike) : Constant  Value=systemP
  Constant10 : Constant  Value=sigma_r
  Constant11 : Constant  Value=channel
  Constant12 : Constant  Value=channel
  Constant13 : Constant  Value=vard
  Constant{14..15,18,25} (4 alike) : Constant  Value=vardq
  Constant{5,16,20,26} (4 alike) : Constant  Value=varq
  Constant17 : Constant  Value=1*1E-2*[2;1]
  Constant2 : Constant  Value=cc
  Constant{6,8,21,29} (4 alike) : Constant  Value=R_k
  Constant22 : Constant  Value=20*1E-2*[2;1]
  Constant23 : Constant  Value=[0.99,0.01;0.01,0.99]
  Constant24 : Constant  Value=sigma_rr
  Constant28 : Constant  Value=vard
  Constant30 : Constant  Value=sigma_pp
  Constant7 : Constant  Value=vard
  Constant9 : Constant  Value=sigma_p
  Data Store Memory : DataStoreMemory  DataStoreName=z  ReadBeforeWriteMsg=warning  WriteAfterWriteMsg=warning  WriteAfterReadMsg=warning  InitialValue=zeros(2,1)  ShowAdditionalParam=off
  Data Store Read : DataStoreRead  DataStoreName=z
  Data Store Read1 : DataStoreRead  DataStoreName=xk
  Data Store Read2 : DataStoreRead  DataStoreName=mkxk
  Data Store Read3 : DataStoreRead  DataStoreName=cxk
  Data Store Write : DataStoreWrite  DataStoreName=observer
  Data Store Write1 : DataStoreWrite  DataStoreName=disturbance  DataStoreElements=disturbance(3:4)
  Data Store Write2 : DataStoreWrite  DataStoreName=z
  Data Store Write3 : DataStoreWrite  DataStoreName=friction
  Data Store Write4 : DataStoreWrite  DataStoreName=mkxk
  Data Store Write5 : DataStoreWrite  DataStoreName=xk
  Data Store Write6 : DataStoreWrite  Commented=on  DataStoreName=immxk
  Data Store Write7 : DataStoreWrite  DataStoreName=immxk
  Data Store Write8 : DataStoreWrite  DataStoreName=cxk
  Display : Display
  Display1 : Display
  MKEKF : MATLAB Function  TreatAsAtomicUnit=on
  MKEKF1 : MATLAB Function  TreatAsAtomicUnit=on
  Multiport Switch : MultiPortSwitch
  Multiport Switch1 : MultiPortSwitch
  Scope{,6,14..15} (4 alike) : Scope  NumInputPorts=2
  Scope1 : Scope  NumInputPorts=3
  Scope{5,10..12,16} (5 alike) : Scope
  Scope13 : Scope  NumInputPorts=3
  Scope2 : Scope  NumInputPorts=4
  Scope3 : Scope  Commented=on
  Scope4 : Scope  Commented=on
  Scope7 : Scope  Commented=on  NumInputPorts=3
  Scope8 : Scope  Commented=on
  Scope9 : Scope  Commented=on  NumInputPorts=3
  command{1,3,9,16,24,27} (6 alike) : DataStoreRead  DataStoreName=position  DataStoreElements=position(3:4)
  command{4..5,10,13,21,23} (6 alike) : DataStoreRead  DataStoreName=velocity  DataStoreElements=velocity(3:4)
  command{6,8,11,14,22,25} (6 alike) : DataStoreRead  DataStoreName=motor_torque  DataStoreElements=motor_torque(3:4)
  command{7,12,15,26} (4 alike) : DataStoreRead  DataStoreName=acceleration  DataStoreElements=acceleration(3:4)
  command17 : DataStoreRead  DataStoreName=xk  DataStoreElements=xk(5:6)
  command18 : DataStoreRead  DataStoreName=mkxk  DataStoreElements=mkxk(3:4)
  command19 : DataStoreRead  DataStoreName=mkxk  DataStoreElements=mkxk(5:6)
  command2 : DataStoreRead  DataStoreName=desired_acc  DataStoreElements=desired_acc(3:4)
  command20 : DataStoreRead  DataStoreName=xk  DataStoreElements=xk(3:4)
  command28 : DataStoreRead  DataStoreName=immxk  DataStoreElements=immxk(1:2)
  computedTorque : MATLAB Function  TreatAsAtomicUnit=on
  disturbance observer : MATLAB Function  TreatAsAtomicUnit=on
  extended kalman filter : MATLAB Function  TreatAsAtomicUnit=on
  extended kalman filter1 : MATLAB Function  Commented=on  TreatAsAtomicUnit=on
  extended kalman filter2 : MATLAB Function  TreatAsAtomicUnit=on
  "process " : MATLAB Function  TreatAsAtomicUnit=on
  process 1 : MATLAB Function  TreatAsAtomicUnit=on
  process 2 : MATLAB Function  TreatAsAtomicUnit=on
  process 3 : MATLAB Function  TreatAsAtomicUnit=on
  wires:
  Constant/1 -> computedTorque/4(para)
  computedTorque/1(y) -> Scope5/1, Data Store Write/1
  Multiport Switch1/1 -> computedTorque/2(dq)
  Multiport Switch/1 -> computedTorque/1(q)
  Constant1/1 -> disturbance observer/5(para)
  command4/1 -> disturbance observer/2(dq)
  command1/1 -> disturbance observer/1(q)
  command6/1 -> disturbance observer/4(cur)
  Data Store Read/1 -> disturbance observer/6(z)
  disturbance observer/2(zz) -> Data Store Write2/1
  disturbance observer/1(TT) -> Scope/2
  command7/1 -> disturbance observer/3(ddq)
  Constant2/1 -> disturbance observer/7(c)
  computedTorque/2(f) -> Data Store Write3/1
  command8/1 -> Scope/1
  command10/1 -> extended kalman filter/2(dq)
  extended kalman filter/2(d) -> Scope6/1, Scope2/1, Scope1/2  "ekf"
  Constant3/1 -> extended kalman filter/5(para)
  command9/1 -> extended kalman filter/1(q)
  command11/1 -> extended kalman filter/4(cur)
  Data Store Read1/1 -> extended kalman filter/6(xk)
  extended kalman filter/1(xkk) -> Data Store Write5/1
  extended kalman filter/3(D) -> Scope1/3
  command12/1 -> extended kalman filter/3(ddq)
  disturbance observer/3(d) -> Data Store Write1/1, Scope1/1
  Data Store Read2/1 -> MKEKF/6(xk)
  Constant4/1 -> MKEKF/5(para)
  command14/1 -> MKEKF/4(cur)
  command15/1 -> MKEKF/3(ddq)
  command13/1 -> MKEKF/2(dq)
  command16/1 -> MKEKF/1(q)
  MKEKF/1(xkk) -> Data Store Write4/1
  MKEKF/2(d) -> Scope2/2  "mkckf"
  MKEKF/4(num) -> Display/1
  Constant6/1 -> extended kalman filter/8(R_k)
  "process "/1(Q_k) -> extended kalman filter/7(Q_k)
  Constant8/1 -> MKEKF/9(R_k)
  Constant9/1 -> MKEKF/10(sigma_p)
  Constant10/1 -> MKEKF/11(sigma_r)
  command3/1 -> Multiport Switch/2
  command5/1 -> Multiport Switch1/2
  command17/1 -> Multiport Switch/3
  command19/1 -> Multiport Switch/4
  command20/1 -> Multiport Switch1/3
  command18/1 -> Multiport Switch1/4
  Constant11/1 -> Multiport Switch/1
  Constant12/1 -> Multiport Switch1/1
  command2/1 -> computedTorque/3(ddq)
  Constant13/1 -> "process "/1(vard)
  Constant5/1 -> "process "/3(varq)
  Constant14/1 -> "process "/2(vardq)
  Constant7/1 -> process 1/1(vard)
  Constant16/1 -> process 1/3(varq)
  Constant15/1 -> process 1/2(vardq)
  process 1/1(Q_k) -> MKEKF/7(Q_k)
  Constant20/1 -> process 2/4(varq)
  Constant18/1 -> process 2/3(vardq)
  Constant17/1 -> process 2/1(vard1)
  Constant21/1 -> extended kalman filter2/7(Rk), extended kalman filter1/7(Rk)
  command22/1 -> extended kalman filter2/3(cur), extended kalman filter1/3(cur)
  command21/1 -> extended kalman filter2/2(dq), extended kalman filter1/2(dq)
  Constant19/1 -> extended kalman filter2/4(para), extended kalman filter1/4(para)
  command24/1 -> extended kalman filter2/1(q), extended kalman filter1/1(q)
  Constant22/1 -> process 2/2(vard2)
  Constant23/1 -> extended kalman filter2/8(T), extended kalman filter1/8(T)
  extended kalman filter1/1(xkk) -> Scope9/1, Data Store Write6/1
  extended kalman filter1/4(d) -> Scope7/1
  extended kalman filter1/6(mu) -> Scope8/1
  extended kalman filter1/5(GAMMA) -> Scope4/1
  process 2/1(Q_k1) -> extended kalman filter2/5(Qk1), extended kalman filter1/5(Qk1)
  process 2/2(Q_k2) -> extended kalman filter2/6(Qk2), extended kalman filter1/6(Qk2)
  extended kalman filter1/7(Pkdiag) -> Scope3/1
  extended kalman filter1/3(xkk2) -> Scope9/3
  extended kalman filter1/2(xkk1) -> Scope9/2
  extended kalman filter2/7(v1v2) -> Scope10/1
  extended kalman filter2/6(mu) -> Scope12/1
  extended kalman filter2/5(GAMMA) -> Scope11/1
  extended kalman filter2/3(xkk2) -> Scope13/3
  extended kalman filter2/2(xkk1) -> Scope13/2
  extended kalman filter2/1(xkk) -> Data Store Write7/1, Scope13/1  "imm"
  extended kalman filter2/4(d) -> Scope6/2  "imm"
  extended kalman filter2/8(PKK1) -> Scope14/1
  extended kalman filter2/9(PKK2) -> Scope14/2
  extended kalman filter2/10(Qkk1) -> Scope15/1
  extended kalman filter2/11(Qkk2) -> Scope15/2
  process 3/1(Q_k) -> MKEKF1/7(Q_k)
  command26/1 -> MKEKF1/3(ddq)
  command23/1 -> MKEKF1/2(dq)
  MKEKF1/4(num) -> Display1/1
  Constant28/1 -> process 3/1(vard)
  Data Store Read3/1 -> MKEKF1/6(xk)
  Constant30/1 -> MKEKF1/9(sigma_p)
  Constant29/1 -> MKEKF1/8(R_k)
  Constant24/1 -> MKEKF1/10(sigma_r)
  MKEKF1/1(xkk) -> Data Store Write8/1
  Constant25/1 -> process 3/2(vardq)
  command27/1 -> MKEKF1/1(q)
  Constant26/1 -> process 3/3(varq)
  Constant27/1 -> MKEKF1/5(para)
  command25/1 -> MKEKF1/4(cur)
  MKEKF1/2(d) -> Scope2/4  "ckf"
  command28/1 -> Scope2/3
  process 1/2(Q_maxk) -> MKEKF/8(Q_maxk)
  MKEKF/7(vec_recp) -> Scope16/1

== system Exp/Control/Gait Generator ==
  Clock1 : Clock
  Constant2 : Constant  Value=f_gait
  Fcn : Fcn  Expr=u-3
  Gait Generator : MATLAB Function  TreatAsAtomicUnit=on
  Scope : Scope
  Scope1 : Scope
  desired_acc : DataStoreWrite  DataStoreName=desired_acc
  desired_position : DataStoreWrite  DataStoreName=desired_position
  desired_velocity : DataStoreWrite  DataStoreName=desired_velocity
  wires:
  Clock1/1 -> Fcn/1
  Fcn/1 -> Gait Generator/1(t)
  Constant2/1 -> Gait Generator/2(f)
  Gait Generator/2(dgait) -> Scope/1, desired_velocity/1
  Gait Generator/3(ddgait) -> Scope1/1, desired_acc/1
  Gait Generator/1(gait) -> desired_position/1

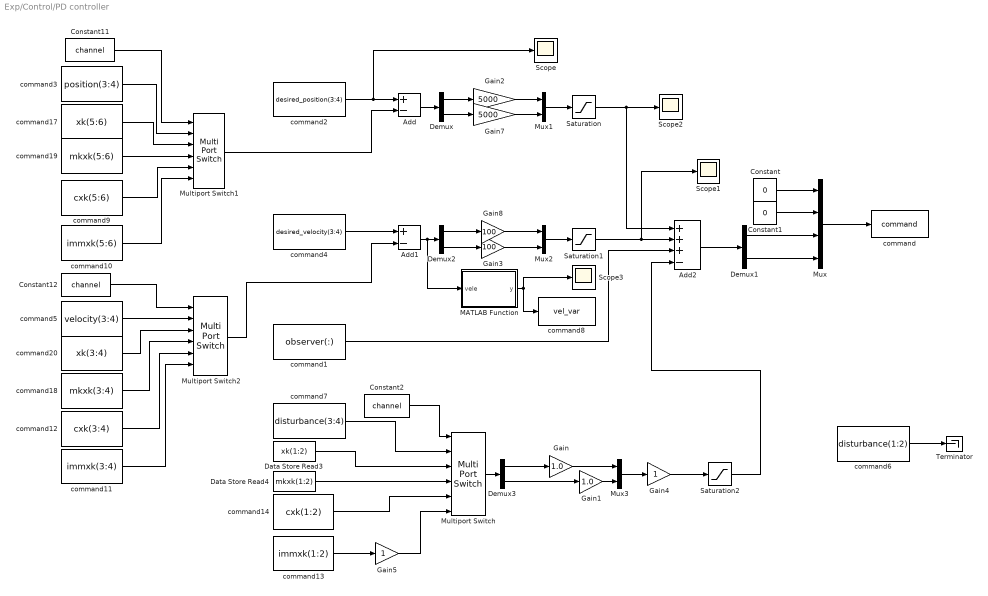
== system Exp/Control/PD controller ==
  Add : Sum  Inputs=+-
  Add1 : Sum  Inputs=+-
  Add2 : Sum  Inputs=+++-
  Constant : Constant  Value=0
  Constant1 : Constant  Value=0
  Constant11 : Constant  Value=channel
  Constant12 : Constant  Value=channel
  Constant2 : Constant  Value=channel
  Data Store Read3 : DataStoreRead  DataStoreName=xk  DataStoreElements=xk(1:2)
  Data Store Read4 : DataStoreRead  DataStoreName=mkxk  DataStoreElements=mkxk(1:2)
  Demux{,1..3} (4 alike) : Demux  Outputs=2
  Gain : Gain  Gain=1.0
  Gain1 : Gain  Gain=1.0
  Gain2 : Gain  Gain=5000
  Gain3 : Gain  Gain=100
  Gain4 : Gain
  Gain5 : Gain
  Gain7 : Gain  Gain=5000
  Gain8 : Gain  Gain=100
  MATLAB Function : MATLAB Function  TreatAsAtomicUnit=on
  Multiport Switch : MultiPortSwitch  Inputs=5
  Multiport Switch1 : MultiPortSwitch  Inputs=5
  Multiport Switch2 : MultiPortSwitch  Inputs=5
  Mux : Mux
  Mux1 : Mux  Inputs=2
  Mux2 : Mux  Inputs=2
  Mux3 : Mux  Inputs=2
  Saturation : Saturate  UpperLimit=50  LowerLimit=-50
  Saturation1 : Saturate  UpperLimit=50  LowerLimit=-50
  Saturation2 : Saturate  UpperLimit=150  LowerLimit=-150
  Scope{,1..3} (4 alike) : Scope
  Terminator : Terminator
  command : DataStoreWrite  DataStoreName=command
  command1 : DataStoreRead  DataStoreName=observer  DataStoreElements=observer(:)
  command10 : DataStoreRead  DataStoreName=immxk  DataStoreElements=immxk(5:6)
  command11 : DataStoreRead  DataStoreName=immxk  DataStoreElements=immxk(3:4)
  command12 : DataStoreRead  DataStoreName=cxk  DataStoreElements=cxk(3:4)
  command13 : DataStoreRead  DataStoreName=immxk  DataStoreElements=immxk(1:2)
  command14 : DataStoreRead  DataStoreName=cxk  DataStoreElements=cxk(1:2)
  command17 : DataStoreRead  DataStoreName=xk  DataStoreElements=xk(5:6)
  command18 : DataStoreRead  DataStoreName=mkxk  DataStoreElements=mkxk(3:4)
  command19 : DataStoreRead  DataStoreName=mkxk  DataStoreElements=mkxk(5:6)
  command2 : DataStoreRead  DataStoreName=desired_position  DataStoreElements=desired_position(3:4)
  command20 : DataStoreRead  DataStoreName=xk  DataStoreElements=xk(3:4)
  command3 : DataStoreRead  DataStoreName=position  DataStoreElements=position(3:4)
  command4 : DataStoreRead  DataStoreName=desired_velocity  DataStoreElements=desired_velocity(3:4)
  command5 : DataStoreRead  DataStoreName=velocity  DataStoreElements=velocity(3:4)
  command6 : DataStoreRead  DataStoreName=disturbance  DataStoreElements=disturbance(1:2)
  command7 : DataStoreRead  DataStoreName=disturbance  DataStoreElements=disturbance(3:4)
  command8 : DataStoreWrite  DataStoreName=vel_var
  command9 : DataStoreRead  DataStoreName=cxk  DataStoreElements=cxk(5:6)
  wires:
  command4/1 -> Add1/1
  Mux/1 -> command/1
  Add2/1 -> Demux1/1
  Demux1/2 -> Mux/4
  Demux1/1 -> Mux/3
  command2/1 -> Scope/1, Add/1
  Constant1/1 -> Mux/2
  Constant/1 -> Mux/1
  command1/1 -> Add2/3
  Add/1 -> Demux/1
  Demux/2 -> Gain7/1
  Demux/1 -> Gain2/1
  Gain2/1 -> Mux1/1
  Gain7/1 -> Mux1/2
  Add1/1 -> MATLAB Function/1(vele), Demux2/1
  Demux2/2 -> Gain3/1
  Demux2/1 -> Gain8/1
  Gain8/1 -> Mux2/1
  Gain3/1 -> Mux2/2
  Mux2/1 -> Saturation1/1
  Mux1/1 -> Saturation/1
  Mux3/1 -> Gain4/1
  command7/1 -> Multiport Switch/2
  Multiport Switch/1 -> Demux3/1
  Demux3/1 -> Gain/1
  Gain/1 -> Mux3/1
  Demux3/2 -> Gain1/1
  Gain1/1 -> Mux3/2
  Gain4/1 -> Saturation2/1
  Data Store Read3/1 -> Multiport Switch/3
  Data Store Read4/1 -> Multiport Switch/4
  Saturation/1 -> Scope2/1, Add2/1
  Saturation1/1 -> Add2/2, Scope1/1
  Constant2/1 -> Multiport Switch/1
  command3/1 -> Multiport Switch1/2
  command5/1 -> Multiport Switch2/2
  command18/1 -> Multiport Switch2/4
  command19/1 -> Multiport Switch1/4
  command20/1 -> Multiport Switch2/3
  Constant12/1 -> Multiport Switch2/1
  command17/1 -> Multiport Switch1/3
  Constant11/1 -> Multiport Switch1/1
  Multiport Switch2/1 -> Add1/2
  Multiport Switch1/1 -> Add/2
  Saturation2/1 -> Add2/4
  command6/1 -> Terminator/1
  MATLAB Function/1(y) -> command8/1, Scope3/1
  command9/1 -> Multiport Switch1/5
  command10/1 -> Multiport Switch1/6
  command12/1 -> Multiport Switch2/5
  command11/1 -> Multiport Switch2/6
  command14/1 -> Multiport Switch/5
  command13/1 -> Gain5/1
  Gain5/1 -> Multiport Switch/6

== matlab function Exp/Control/Feedforward&nonlinearFeekbackLinearlization&Observer/computedTorque ==
  data: q input; y output; dq input; ddq input; para input; f output
function [y,f]= fcn(q,dq,ddq,para)

l1=0.42;
tau_c2=para(1);
tau_s2=para(2);
dqs2=para(3);
eta2=para(4);
X2=para(5);
Y2=para(6);
J2=para(7);

tau_c1=para(8);
tau_s1=para(9);
dqs1=para(10);
eta1=para(11);
X1=para(12);
Y1=para(13);
J1=para(14);

T1=(J1+2*l1*(X2*cos(q(2))-Y2*sin(q(2)))).*ddq(1)+(J2+l1*(X2*cos(q(2))-Y2*sin(q(2)))).*ddq(2)...
    -l1*(X2*sin(q(2))+Y2*cos(q(2))).*(2*dq(1).*dq(2)+dq(2).*dq(2))+...
    +9.7925*(X1*sin(q(1))+Y1*cos(q(1)+X2*sin(q(1)+q(2))+Y2*cos(q(1)+q(2))))+...
    0;
%     (tau_c1+(tau_s1-tau_c1)*exp(-dq(1)/dqs1)).*customSIGN(dq(1))+eta1*dq(1);

T2=(J2+l1*(X2*cos(q(2))-Y2*sin(q(2)))).*ddq(1)+J2.*ddq(2)+l1*(X2*sin(q(2))+Y2*cos(q(2))).*dq(1).*dq(1)...
    +9.7925*(X2*sin(q(1)+q(2))+Y2*cos(q(1)+q(2)))+...
    0;
%     (tau_c2+(tau_s2-tau_c2)*exp(-dq(2)/dqs2)).*customSIGN(dq(2))+eta2*dq(2);

y = [T1,T2];


f1=(tau_c1+(tau_s1-tau_c1)*exp(-dq(1)/dqs1)).*customSIGN(dq(1))+eta1*dq(1);
f2=(tau_c2+(tau_s2-tau_c2)*exp(-dq(2)/dqs2)).*customSIGN(dq(2))+eta2*dq(2);

f=[f1,f2];
end



function y=customSIGN(u)
threshold=0.05;
if(u>threshold)
    y=1;
elseif(u<-threshold)
    y=-1;
else
    y=u/threshold;
end


end

== matlab function Exp/Position/MATLAB Function ==
  data: time input; Bias input; y input; y output; Bias output
function [y, Bias] = fcn(time, Bias, y)

if time <= 3
    Bias=y;
    y=y*0;
else
    y=y-Bias;
end

end

== matlab function Exp/6 Axis Force//Torque Sensor/MATLAB Function1 ==
  data: F input; d1 output; theta input; d2 output
function [d1,d2] = fcn(F,theta)


% disturbance measurement
delta1=0.285;
delta2=0.235;
l1=0.42;
% 
Fx1=-F(3);
Fy1=-F(4);
Fx2=-F(1);
Fy2=-F(2);
%
d2=-Fx2*delta2;
%
idot=sqrt(delta2^2+l1^2-2*delta2*l1*cos(pi+theta));
phi=pi/2-acos((idot^2+delta2^2-l1^2)/(2*idot*delta2));

d1=-Fx2*sin(phi)*idot-Fy2*cos(phi)*idot-Fx1*delta1;

end

== matlab function Exp/6 Axis Force//Torque Sensor/MATLAB Function2 ==
  data: F input; F_cor output; q input
function F_cor = fcn(F,q)


hipx=F(3);
hipy=F(4);
kneex=F(1);
kneey=F(2);

hip =q(1);
knee=q(1)+q(2);

hipx_=-2.826*hip -0.144;
hipy_= 1.71*hip^2-0.07893*hip -0.02702;

kneex_= -2.567*knee+0.1642;
kneey_= 1.311*knee^2+ 0.08684*knee -0.04121;



F_cor=[kneex-kneex_,kneey-kneey_,hipx-hipx_,hipy-hipy_];
